simulink model "modelo_serial(el utilizado)"  (R2019a)
settings: Solver=FixedStepAuto  StartTime=0.0  StopTime=inf  RelTol=1e-3  EnableMultiTasking=on
undefined symbols (not defined in the file): serial
libraries: simulink x3, instrumentlib x3
settings Model: ExtModeTrigDuration=2  Creator=Kike  LastModifiedBy=Kike
settings SolverCC: AutoInsertRateTranBlk=on
settings OptimizationCC: EnhancedBackFolding=on  PassReuseOutputArgsAs=Individual arguments  MaxStackSize=64  OptimizeBlockOrder=speed  DifferentSizesBufferReuse=on
settings DebuggingCC: ParameterTunabilityLossMsg=error
settings HardwareCC: ProdBitPerInt=16  ProdBitPerPointer=16  ProdBitPerSizeT=16  ProdBitPerPtrDiffT=16  ProdLargestAtomicFloat=None  ProdWordSize=8  ProdHWDeviceType=Atmel->AVR
settings SFSimCC: MATLABDynamicMemAlloc=off
settings RTWCC: SystemTargetFile=ert.tlc  HardwareBoard=Arduino Nano 3.0  TLCOptions=-aInlineSetEventsForThisBaseRateFcn=TLC_FALSE -aSuppressMultiTaskScheduler=TLC_FALSE -aRateBasedStepFcn=1  TemplateMakefile=ert_default_tmf  GenerateReport=on  Toolchain=Arduino AVR  BuildConfiguration=Faster Runs  IncludeHyperlinkInReport=on  LaunchReport=on  GenerateTraceInfo=on  GenerateTraceReport=on  GenerateTraceReportSl=on  GenerateTraceReportSf=on  GenerateTraceReportEml=on
settings CodeAppCC: ForceParamTrailComments=on  IgnoreCustomStorageClasses=off  OperatorAnnotations=on  SimulinkDataObjDesc=on  SFDataObjDesc=on  InsertBlockDesc=on
settings ERTTargetCC: SupportContinuousTime=on  SupportVariableSizeSignals=on  ExtModeStaticAllocSize=250

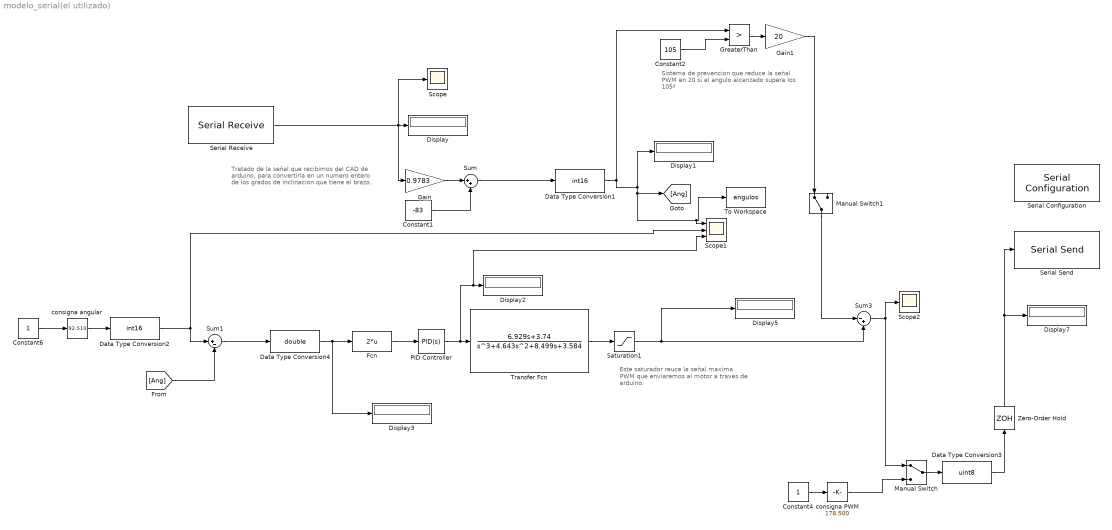
== system modelo_serial(el utilizado) ==
  note: Este saturador reuce la señal maxima
      | PWM que enviaremos al motor a traves
      | de arduino.
  note: Tratado de la señal que recibimos del CAD
      | de arduino, para convertirla en un numero
      | entero de los grados de inclinacion que tiene
      | el brazo.
  note: Sistema de prevencion que reduce la señal
      | PWM en 20 si el angulo alcanzado supera
      | los 105º
  Constant1 : Constant  Value=-83
  Constant2 : Constant  Value=105  OutDataTypeStr=int16
  Constant4 : Constant
  Constant6 : Constant
  Data Type Conversion1 : DataTypeConversion  OutDataTypeStr=int16
  Data Type Conversion2 : DataTypeConversion  OutDataTypeStr=int16
  Data Type Conversion3 : DataTypeConversion  OutDataTypeStr=uint8
  Data Type Conversion4 : DataTypeConversion  OutDataTypeStr=double
  Display{,1..3,5,7} (6 alike) : Display
  Fcn : Fcn  Expr=2*u
  Gain : Gain  Gain=0.9783
  Gain1 : Gain  Gain=20
  GreaterThan : RelationalOperator  Operator=>  OutDataTypeStr=boolean  RndMeth=Simplest
  Manual Switch : ManualSwitch
  Manual Switch1 : ManualSwitch
  PID Controller : simulink/Continuous/PID Controller  Controller=PID  Form=Ideal  TimeDomain=Continuous-time  SampleTime=-1  IntegratorMethod=Forward Euler  FilterMethod=Forward Euler  ControllerParametersSource=internal  P=0.180391749835672  I=1.76614508523059  D=0  UseFilter=on  N=100  TunerSelectOption=Transfer Function Based (PID Tuner App)  InitialConditionSource=internal  InitialConditionForIntegrator=0  InitialConditionForFilter=0  DifferentiatorICPrevScaledInput=0  ExternalReset=none  TrackingMode=off  Kt=1  LimitOutput=off  UpperSaturationLimit=inf  LowerSaturationLimit=-inf  LinearizeAsGain=on  AntiWindupMode=clamping  Kb=1  POutMin=[]  POutMax=[]  IOutMin=[]  IOutMax=[]  DOutMin=[]  DOutMax=[]  NOutMin=[]  NOutMax=[]  SumOutMin=[]  SumOutMax=[]  SaturationOutMin=[]  SaturationOutMax=[]  PParamMin=[]  PParamMax=[]  IParamMin=[]  IParamMax=[]  DParamMin=[]  DParamMax=[]  NParamMin=[]  NParamMax=[]  KbParamMin=[]  KbParamMax=[]  KtParamMin=[]  KtParamMax=[]  KbOutMin=[]  KbOutMax=[]  KtOutMin=[]  KtOutMax=[]  IntegratorOutMin=[]  IntegratorOutMax=[]  FilterOutMin=[]  FilterOutMax=[]  SumI1OutMin=[]  SumI1OutMax=[]  SumI2OutMin=[]  SumI2OutMax=[]  SumI3OutMin=[]  SumI3OutMax=[]  SumI4OutMin=[]  SumI4OutMax=[]  SumDOutMin=[]  SumDOutMax=[]  DifferentiatorOutMin=[]  DifferentiatorOutMax=[]  FilterDiffOutCoefMin=[]  FilterDiffOutCoefMax=[]  ReciprocalOutMin=[]  ReciprocalOutMax=[]  SumDenOutMin=[]  SumDenOutMax=[]  SumNumOutMin=[]  SumNumOutMax=[]  DivideOutMin=[]  DivideOutMax=[]  IntegratorContinuousStateAttributes=''  IntegratorStateMustResolveToSignalObject=off  IntegratorRTWStateStorageClass=Auto  FilterContinuousStateAttributes=''  FilterStateMustResolveToSignalObject=off  FilterRTWStateStorageClass=Auto  ParallelPVariant=Passthrough  IdealPVariant=InternalParameters  IVariant=InternalParameters  DVariant=InternalParameters  IntegratorVariant=Continuous  SatVariant=Disabled  AWVariant=Passthrough  PCopyVariant=Disabled  TRVariant=Disabled  FdbkBlocksVariant=Forward  IdealPFdbkVariant=Disabled  SatFdbkVariant=Disabled  DerivativeFilterVariant=ContFilter  NVariant=InternalParameters  NCopyVariant=Disabled  FilterICVariant=InternalICsFilter  IntegratorICVariant=InternalICs  ExternalResetVariant=Disabled  TRSumVariant=Passthrough  SumFdbkVariant=Disabled  SumVariant=Sum_PID
  Saturation1 : Saturate  UpperLimit=255  LowerLimit=0
  Scope : Scope
  Scope1 : Scope  NumInputPorts=3
  Scope2 : Scope
  Serial Configuration : instrumentlib/Serial Configuration  Priority=-200000  ComPortMenu=<Please select a port...>  ComPort=COM9  ObjConstructor=serial('COM9');  BaudRate=115200  DataBits=8  Parity=none  StopBits=1  FlowControl=none  Timeout=10  ByteOrder=LittleEndian
  Serial Receive : instrumentlib/Serial Receive  ComPortMenu=<Please select a port...>  ComPort=COM9  ObjConstructor=serial('COM9');  Terminator=<none>  DataSize=1  DataType=uint8  EnableBlockingMode=on  ActionDataUnavailable=Output last received value  CustomValue=0  SampleTime=0.01
  Serial Send : instrumentlib/Serial Send  ComPortMenu=<Please select a port...>  ComPort=COM9  ObjConstructor=serial('COM9');  Terminator=<none>  EnableBlockingMode=on
  Sum : Sum  Inputs=|++
  Sum1 : Sum  Inputs=|+-
  Sum3 : Sum  Inputs=|-+
  To Workspace : ToWorkspace  VariableName=angulos  SaveFormat=Structure With Time  SampleTime=0.05
  Transfer Fcn : TransferFcn  Numerator=[6.929 3.74]  Denominator=[1 4.643 8.499 3.584]
  Zero-Order Hold : ZeroOrderHold  SampleTime=0.01
  consigna PWM : simulink/Math Operations/Slider Gain  gain=178.500  low=0  high=255
  "consigna angular " : simulink/Math Operations/Slider Gain  gain=92.510  low=12  high=95
  wires:
  "consigna angular "/1 -> Data Type Conversion2/1
  Constant1/1 -> Sum/2
  PID Controller/1 -> Scope1/3, Display2/1, Transfer Fcn/1
  Gain/1 -> Sum/1
  Data Type Conversion2/1 -> Scope1/2, Sum1/1
  [Ang] -> Sum1/2
  Manual Switch/1 -> Data Type Conversion3/1
  Constant4/1 -> consigna PWM/1
  consigna PWM/1 -> Manual Switch/2
  Zero-Order Hold/1 -> Serial Send/1, Display7/1
  Serial Receive/1 -> Scope/1, Display/1, Gain/1
  Sum/1 -> Data Type Conversion1/1
  Data Type Conversion1/1 -> To Workspace/1, Scope1/1, [Ang], Display1/1, GreaterThan/1
  Data Type Conversion3/1 -> Zero-Order Hold/1
  Constant2/1 -> GreaterThan/2
  Transfer Fcn/1 -> Saturation1/1
  Sum3/1 -> Manual Switch/1, Scope2/1
  GreaterThan/1 -> Gain1/1
  Constant6/1 -> "consigna angular "/1
  Manual Switch1/1 -> Sum3/1
  Gain1/1 -> Manual Switch1/1
  Sum1/1 -> Data Type Conversion4/1
  Data Type Conversion4/1 -> Display3/1, Fcn/1
  Fcn/1 -> PID Controller/1
  Saturation1/1 -> Sum3/2, Display5/1
